simulink model "TrafficLight_StateFlow"  (R2018b)
settings: Solver=FixedStepDiscrete  StartTime=0.0  StopTime=inf  RelTol=1e-3
settings Model: Creator=ayamu  LastModifiedBy=ayamu
settings OptimizationCC: DefaultParameterBehavior=Inlined  EnhancedBackFolding=on  PassReuseOutputArgsAs=Individual arguments  OptimizeBlockOrder=speed  DifferentSizesBufferReuse=on  OptimizationCustomize=off
settings DebuggingCC: UnderspecifiedInitializationDetection=Classic  MergeDetectMultiDrivingBlocksExec=none  ParameterTunabilityLossMsg=error
settings ModelReferenceCC: PropagateSignalLabelsOutOfModel=off
settings SFSimCC: MATLABDynamicMemAlloc=off
settings RTWCC: SystemTargetFile=ert.tlc  GenCodeOnly=on  TemplateMakefile=ert_default_tmf  GenerateReport=on  IncludeHyperlinkInReport=on  LaunchReport=on  GenerateTraceInfo=on  GenerateTraceReport=on  GenerateTraceReportSl=on  GenerateTraceReportSf=on  GenerateTraceReportEml=on
settings CodeAppCC: ForceParamTrailComments=on  IgnoreCustomStorageClasses=off  OperatorAnnotations=on  SimulinkDataObjDesc=on  SFDataObjDesc=on  InsertBlockDesc=on
settings ERTTargetCC: TargetLangStandard=C99 (ISO)  GenerateSampleERTMain=on  InlinedParameterPlacement=NonHierarchical  ERTCustomFileTemplate=example_file_process.tlc

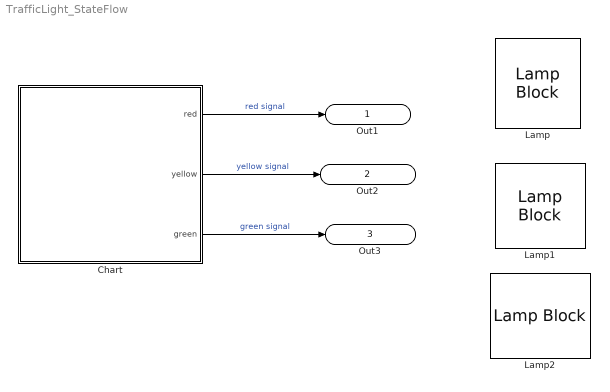
== system TrafficLight_StateFlow ==
  Chart : Stateflow chart  TreatAsAtomicUnit=on
  Lamp : LampBlock  WebBlockId=2
  Lamp1 : LampBlock  WebBlockId=3
  Lamp2 : LampBlock  WebBlockId=4
  Out1 : Outport
  Out2 : Outport  Port=2
  Out3 : Outport  Port=3  SignalName=green signal
  wires:
  Chart/1(red) -> Out1/1  "red signal"
  Chart/2(yellow) -> Out2/1  "yellow signal"
  Chart/3(green) -> Out3/1  "green signal"

== stateflow chart TrafficLight_StateFlow/Chart ==
  state Ready_
    en:
    red = uint8(0);
    yellow = uint8(0);
    green = uint8(0);
    du:
    red = uint8(0);
    yellow = uint8(1);
    green = uint8(0);
    ex:
  state Stop_
    en:
    red = uint8(0);
    yellow = uint8(0);
    green = uint8(0);
    du:
    red = uint8(1);
    yellow = uint8(0);
    green = uint8(0);
    ex:
  state Go_
    en:
    red = uint8(0);
    yellow = uint8(0);
    green = uint8(0);
    du:
    red = uint8(0);
    yellow = uint8(0);
    green = uint8(1);
    ex:
  (default) -> Stop_
  Stop_ -> Ready_ : after(3000,msec)
  Go_ -> Stop_ : after(3000,msec)
  Ready_ -> Go_ : after(3000,msec)
  data: red output uint8; yellow output uint8; green output uint8
